simulink model "rover_open_loop"  (R2021a)
settings: Solver=VariableStepAuto  StartTime=0.0  StopTime=50  RelTol=1e-3
InitFcn:
  | m = 1025;
  | g = -9.807;
  | r = 0.25;
  | Im = 1;
  | l1 = 2;
  | lB = 1;
  | l2 = 1;
  | l3 = 1;
  | gamma = pi/2;
  | beta = pi/2;
settings Model: Creator=giuse  LastModifiedBy=giuse
settings SolverCC: AlgebraicLoopSolver=TrustRegion
settings DebuggingCC: SFMachineParentedDataDiag=warning

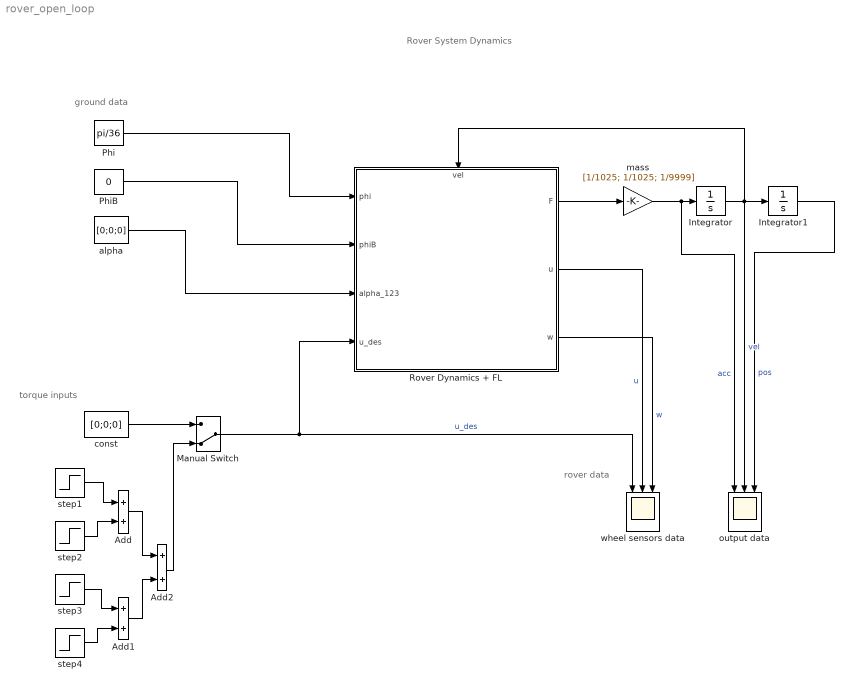
== system rover_open_loop ==
  note: Rover System Dynamics
  note: torque inputs
  note: rover data
  note: ground data
  Add : Sum
  Add1 : Sum
  Add2 : Sum
  Integrator : Integrator
  Integrator1 : Integrator
  Manual Switch : ManualSwitch  CurrentSetting=0
  Phi : Constant  Value=pi/36
  PhiB : Constant  Value=0
  Rover Dynamics + FL : Subsystem
      settings: PortSchema="{\"entries\":[{\"content\":{\"sides\":[{\"content\":{\"connectorIds\":[\"In1\",\"In2\",\"In3\",\"In4\"]},\"type\":\"ConnectorPlacement.EquallySpacedRectSide\",\"uuid\":\"f208f17f-8746-4e0c-80bc-5c26f9d80af4\"},{\"content\":{\"connectorIds\":[\"Out1\",\"Out2\",\"Out3\"],\"side\":\"RIGHT\"},\"type\":\"ConnectorPlacement.EquallySpacedRectSide\",\"uuid\":\"c07668f0-5ba0-4e78-91b8-46ca16e4b345\"},{\"content\":{\"connectorIds\":[\"In5\"],\"side\":\"TOP\"},\"type\":\"ConnectorPlacement.EquallySpacedRectSide\",\"uuid\":\"b9fd77b4-78ae-4ae2-b227-fcaa8ed91b9e\"}]},\"type\":\"ConnectorPlacement.EquallySpacedConnector\",\"uuid\":\"f0e3a283-04fe-443c-8a96-769d22dcf24d\"}],\"packageUris\":[\"http://schema.mathworks.com/mf0/Connector/R2020b\"],\"version\":\"1.0\"}"
  alpha : Constant  Value=[0;0;0]
  const : Constant  Value=[0;0;0]
  mass : Gain  Gain=[1/1025; 1/1025; 1/9999]
  output data : Scope  NumInputPorts=3
  step1 : Step  Time=5  Before=[0;0;0]  After=[-100;-100;-100]  SampleTime=0
  step2 : Step  Time=20  Before=[0;0;0]  After=[100;100;100]  SampleTime=0
  step3 : Step  Time=20  Before=[0;0;0]  After=[100; 100; 100]  SampleTime=0
  step4 : Step  Time=35  Before=[0;0;0]  After=[-100;-100;-100]  SampleTime=0
  wheel sensors data : Scope  NumInputPorts=3
  wires:
  Integrator/1 -> Integrator1/1, Rover Dynamics + FL/5(vel), output data/2  "vel"
  Integrator1/1 -> output data/3  "pos"
  step1/1 -> Add/1
  step2/1 -> Add/2
  Add/1 -> Add2/1
  mass/1 -> Integrator/1, output data/1  "acc"
  const/1 -> Manual Switch/1
  Manual Switch/1 -> wheel sensors data/1, Rover Dynamics + FL/4(u_des)  "u_des"
  Phi/1 -> Rover Dynamics + FL/1(phi)
  PhiB/1 -> Rover Dynamics + FL/2(phiB)
  alpha/1 -> Rover Dynamics + FL/3(alpha_123)
  Rover Dynamics + FL/1(F) -> mass/1
  Rover Dynamics + FL/2(u) -> wheel sensors data/2  "u"
  Rover Dynamics + FL/3(w) -> wheel sensors data/3  "w"
  step4/1 -> Add1/2
  step3/1 -> Add1/1
  Add1/1 -> Add2/2
  Add2/1 -> Manual Switch/2

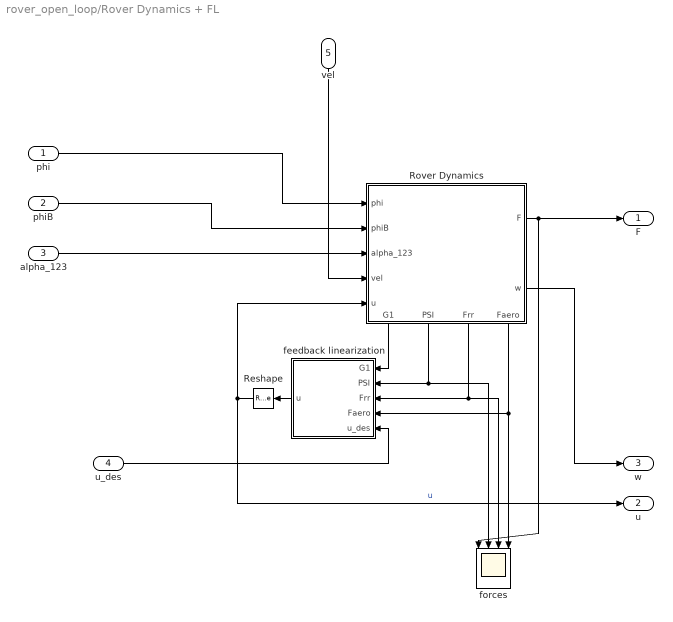
== system rover_open_loop/Rover Dynamics + FL ==
  phi : Inport
  phiB : Inport  Port=2
  alpha_123 : Inport  Port=3
  u_des : Inport  Port=4
  vel : Inport  Port=5
  Reshape : Reshape  OutputDimensionality=Customize  OutputDimensions=[3,1]
  Rover Dynamics : Subsystem
      settings: PortSchema="{\"entries\":[{\"content\":{\"sides\":[{\"content\":{\"connectorIds\":[\"In1\",\"In2\",\"In3\",\"In4\",\"In5\"]},\"type\":\"ConnectorPlacement.EquallySpacedRectSide\",\"uuid\":\"2c5c2f99-3707-47c3-a329-65b8e339adb8\"},{\"content\":{\"connectorIds\":[\"Out1\",\"Out2\"],\"side\":\"RIGHT\"},\"type\":\"ConnectorPlacement.EquallySpacedRectSide\",\"uuid\":\"f105f459-3128-4cb9-820e-42fcacb4be44\"},{\"content\":{\"connectorIds\":[],\"side\":\"TOP\"},\"type\":\"ConnectorPlacement.EquallySpacedRectSide\",\"uuid\":\"039f917f-aa40-46c7-97c6-4866e73dc8bf\"},{\"content\":{\"connectorIds\":[\"Out3\",\"Out4\",\"Out5\",\"Out6\"],\"side\":\"BOTTOM\"},\"type\":\"ConnectorPlacement.EquallySpacedRectSide\",\"uuid\":\"c5311cab-bdc5-46a6-8708-11314025c569\"}]},\"type\":\"ConnectorPlacement.EquallySpacedConnector\",\"uuid\":\"7d99694d-f908-4009-add1-c665530a1a7a\"}],\"packageUris\":[\"http://schema.mathworks.com/mf0/Connector/R2020b\"],\"version\":\"1.0\"}"
  feedback linearization : MATLAB Function  TreatAsAtomicUnit=on
  forces : Scope  NumInputPorts=4
  F : Outport
  u : Outport  Port=2
  w : Outport  Port=3
  wires:
  Rover Dynamics/4(PSI) -> forces/2, feedback linearization/2(PSI)
  Rover Dynamics/1(F) -> forces/1, F/1
  alpha_123/1 -> Rover Dynamics/3(alpha_123)
  phiB/1 -> Rover Dynamics/2(phiB)
  u_des/1 -> feedback linearization/5(u_des)
  feedback linearization/1(u) -> Reshape/1
  Rover Dynamics/5(Frr) -> forces/3, feedback linearization/3(Frr)
  Reshape/1 -> Rover Dynamics/5(u), u/1  "u"
  Rover Dynamics/2(w) -> w/1
  phi/1 -> Rover Dynamics/1(phi)
  vel/1 -> Rover Dynamics/4(vel)
  Rover Dynamics/6(Faero) -> feedback linearization/4(Faero), forces/4
  Rover Dynamics/3(G1) -> feedback linearization/1(G1)

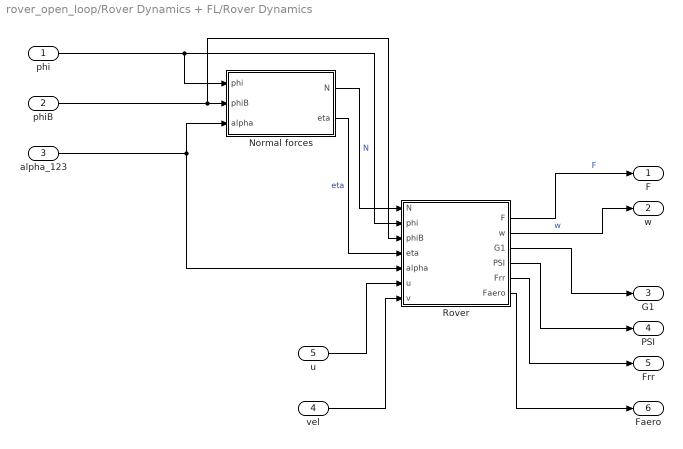
== system rover_open_loop/Rover Dynamics + FL/Rover Dynamics ==
  phi : Inport
  phiB : Inport  Port=2
  alpha_123 : Inport  Port=3
  vel : Inport  Port=4
  u : Inport  Port=5
  Normal forces : MATLAB Function  TreatAsAtomicUnit=on
  Rover : MATLAB Function  TreatAsAtomicUnit=on
  F : Outport
  w : Outport  Port=2
  G1 : Outport  Port=3
  PSI : Outport  Port=4
  Frr : Outport  Port=5
  Faero : Outport  Port=6
  wires:
  Rover/1(F) -> F/1  "F"
  phiB/1 -> Normal forces/2(phiB), Rover/3(phiB)
  phi/1 -> Rover/2(phi), Normal forces/1(phi)
  alpha_123/1 -> Rover/5(alpha), Normal forces/3(alpha)
  Normal forces/1(N) -> Rover/1(N)  "N"
  Normal forces/2(eta) -> Rover/4(eta)  "eta"
  vel/1 -> Rover/7(v)
  Rover/2(w) -> w/1  "w"
  u/1 -> Rover/6(u)
  Rover/3(G1) -> G1/1
  Rover/4(PSI) -> PSI/1
  Rover/5(Frr) -> Frr/1
  Rover/6(Faero) -> Faero/1

== matlab function rover_open_loop/Rover Dynamics + FL/Rover Dynamics/Rover ==
  data: N input; phi input; phiB input; eta input; alpha input; F output; u input; v input; w output; G1 output; PSI output; Frr output; Faero output
function [F, w, G1, PSI, Frr, Faero] = dyn(N, phi, phiB, eta, alpha, u, v)

r = 0.25;   % wheel radius

c1 = cos(alpha(1));
c2 = cos(alpha(2));
c3 = cos(alpha(3));
s1 = sin(alpha(1));
s2 = sin(alpha(2));
s3 = sin(alpha(3));


%% wheel velocities
w_ = norm(v(1:2))/r; 
w = [w_; w_; w_]


%% input matrix
G = [-(1/r)*c1, -(1/r)*c2, -(1/r)*c3;
        (1/r)*s1, (1/r)*s2, (1/r)*s3;
        -(1/r)*eta(1), 0, 0];
G1 = G(1,:);

%% torque/force components due to gravity
R = [cos(phi) -sin(phi) 0; sin(phi) cos(phi) 0; 0 0 1]; % rotation matrix
PSI_ = R*[N(1)*s1 + N(2)*s2 + N(3)*s3;
        N(1)*c1 + N(2)*c2 + N(3)*c3;
        0];
PSI = [PSI_(1); 0; 0]
tau_g = [
    -N(1)*r*sin(phi+alpha(1));
    -N(2)*r*sin(phi+phiB+alpha(2));
    -N(3)*r*sin(phi+phiB+alpha(3))
];

%% torque/force components due to aerodinamic drag
c_aero = 0.2; % not used
Faero = [-c_aero*v(1); -c_aero*v(2); 0];
tau_aero = [norm(Faero)*r; norm(Faero)*r; norm(Faero)*r];

%% torque/force components due to rolling resistance
c_rr = 0.02;  % rolling coefficient
tau_rr = [-c_rr*N(1); -c_rr*N(2); -c_rr*N(3)]
Frr = [(sum(tau_rr))*cos(phi); (sum(tau_rr))*sin(phi); 0];

%% Dynamic model

F_ = G*u + PSI + Faero;

% check rolling resistance
if( norm(v(1:2))<0.1 && abs(norm(F_(1:2)))<=abs(norm(Frr(1:2))) )
    F = [0;0;0];
    Frr = [0;0;0];
else
    F = F_ + Frr;
end






%

== matlab function rover_open_loop/Rover Dynamics + FL/feedback linearization ==
  data: G1 input; u output; PSI input; Frr input; Faero input; u_des input
function u = FL(G1, PSI, Frr, Faero, u_des)

u = [
    u_des(1) - (PSI(1)+Frr(1))/(3*G1(1));
    u_des(2) - (PSI(1)+Frr(1))/(3*G1(2));
    u_des(3) - (PSI(1)+Frr(1))/(3*G1(3))
]

== matlab function rover_open_loop/Rover Dynamics + FL/Rover Dynamics/Normal forces ==
  data: phi input; N output; phiB input; alpha input; eta output
function [N,eta] = normal_forces(phi, phiB, alpha)

% constant data
m = 1025;
g = -9.807;
r = 0.25;
l1 = 2;
lB = 1;
l2 = 1;
l3 = 1;
gamma = pi/2;
beta = pi/2;

% wheel-link angle
theta1 = pi/2 - gamma/2;
thetaB = pi/2 + gamma/2;
theta2 = pi/2 - beta/2;
theta3 = pi/2 + beta/2;

%% ground to pivot vectors
R = [cos(phi) -sin(phi); sin(phi) cos(phi)];
RB = [cos(phiB) -sin(phiB); sin(phiB) cos(phiB)];

a = R*[l1*cos(theta1)-r*sin(alpha(1)); l1*sin(theta1)+r*cos(alpha(1))];
b = R*[lB*cos(thetaB); lB*sin(thetaB)];
c = R*RB*[l2*cos(theta2)-r*sin(alpha(2)); l2*sin(theta2)+r*cos(alpha(2))];
d = R*RB*[l3*cos(theta3)-r*sin(alpha(3)); l3*sin(theta3)+r*cos(alpha(3))];

w = a-b;
eta = [-sin(alpha(1)), cos(alpha(1)); -cos(alpha(1)), -sin(alpha(1))]*w

a_ = abs(a(1));
b_ = abs(b(1));
c_ = abs(c(1));
d_ = abs(d(1));

%% Forces
Fz = m*g;
Fz1 = Fz*(b_/(a_+b_));
FzB = Fz*(a_/(a_+b_));
Fz2 = FzB*(d_/(c_+d_));
Fz3 = FzB*(c_/(c_+d_));

N = [-Fz1; -Fz2; -Fz3]

end
